simulink model "hybrid_ems_p8"  (R2026a)
settings: Solver=ode4  StopTime=604800  FixedStep=3600

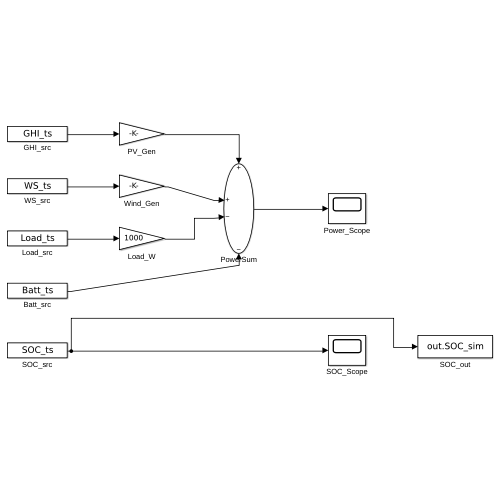
[thumbnail: Simulink's stored preview of the top-level diagram]
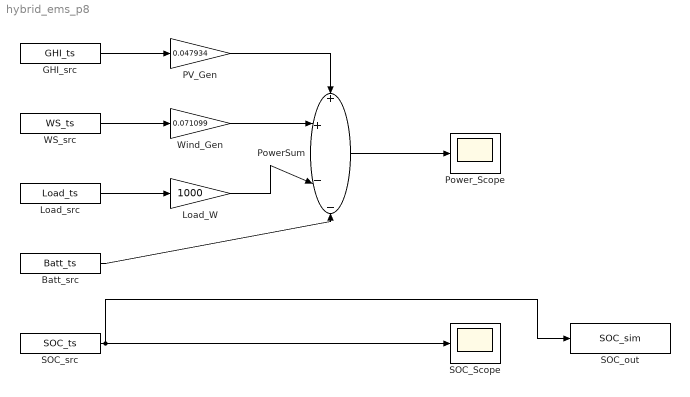
== system hybrid_ems_p8 ==
  Batt_src : FromWorkspace  VariableName=Batt_ts
  GHI_src : FromWorkspace  VariableName=GHI_ts
  Load_W : Gain  Gain=1000
  Load_src : FromWorkspace  VariableName=Load_ts
  PV_Gen : Gain  Gain=0.047934
  PowerSum : Sum  Inputs=++--
  Power_Scope : Scope
  SOC_Scope : Scope
  SOC_out : ToWorkspace  VariableName=SOC_sim  SaveFormat=Timeseries  SampleTime=-1
  SOC_src : FromWorkspace  VariableName=SOC_ts
  WS_src : FromWorkspace  VariableName=WS_ts
  Wind_Gen : Gain  Gain=0.071099
  wires:
  GHI_src/1 -> PV_Gen/1
  WS_src/1 -> Wind_Gen/1
  Load_src/1 -> Load_W/1
  PV_Gen/1 -> PowerSum/1
  Wind_Gen/1 -> PowerSum/2
  Load_W/1 -> PowerSum/3
  Batt_src/1 -> PowerSum/4
  PowerSum/1 -> Power_Scope/1
  SOC_src/1 -> SOC_Scope/1, SOC_out/1
